simulink model "mat_model"  (R2025b)
settings: Solver=VariableStepAuto  StartTime=0.0  StopTime=10.0  RelTol=1e-3
undefined symbols (not defined in the file): c_p, m, Q, T_in, T_ref
settings Model: Creator=marob  LastModifiedBy=marob

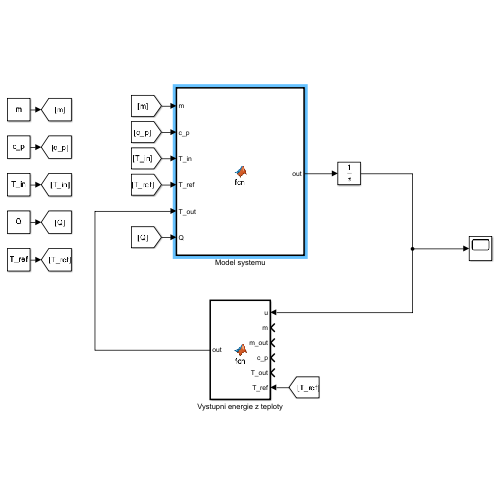
[thumbnail: Simulink's stored preview of the top-level diagram]
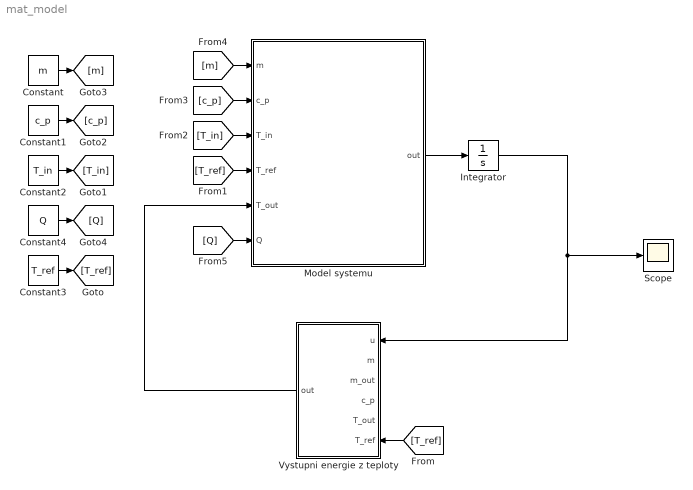
== system mat_model ==
  Constant : Constant  Value=m
  Constant1 : Constant  Value=c_p
  Constant2 : Constant  Value=T_in
  Constant3 : Constant  Value=T_ref
  Constant4 : Constant  Value=Q
  Integrator : Integrator
  Model systemu : MATLAB Function  TreatAsAtomicUnit=on
  Scope : Scope
  Vystupni energie z teploty : MATLAB Function  TreatAsAtomicUnit=on
  wires:
  Model systemu/1(out) -> Integrator/1
  Integrator/1 -> Vystupni energie z teploty/1(u), Scope/1
  [T_ref] -> Vystupni energie z teploty/6(T_ref)
  Constant3/1 -> [T_ref]
  Constant2/1 -> [T_in]
  Constant/1 -> [m]
  Constant1/1 -> [c_p]
  Vystupni energie z teploty/1(out) -> Model systemu/5(T_out)
  [T_ref] -> Model systemu/4(T_ref)
  [T_in] -> Model systemu/3(T_in)
  [c_p] -> Model systemu/2(c_p)
  [m] -> Model systemu/1(m)
  Constant4/1 -> [Q]
  [Q] -> Model systemu/6(Q)

== matlab function mat_model/Vystupni energie z teploty ==
  data: u input; m input; out output; m_out input; c_p input; T_out input; T_ref input
function out = fcn(u,m,m_out,c_p,T_out,T_ref)
out = m_out*c_p*(T_out - T_ref);

== matlab function mat_model/Model systemu ==
  data: m input; out output; c_p input; T_in input; T_ref input; T_out input; Q input
function out = fcn(m,c_p,T_in,T_ref,T_out,Q)
out = (1/(m*c_p)) * (T_in-T_ref)-T_out + Q;
